simulink model "HEV_Ctrl_V1_1"  (R2018a)
settings: configuration reference "Config_Ctrl" (kept outside this file)
PreLoadFcn:
  | HEV_Ctrl_V1_PreLoad
undefined symbols (not defined in the file or in its folder): AstEnblEngSpdMin_H_K, AstEnblEngSpdMin_L_K, AstEnblSocMin_H_K, AstEnblSocMin_L_K, AstEnblVehSpdMin_H_K, AstEnblVehSpdMin_L_K, AstTrqCmpSOC_K2, AstTrqCmpSOC_X, AstTrqDstBase_K3, DifferentialGearRatio_K, DrvReqPropTrq_K3, DrvReqPropTrqMax_K, eHevCtrlMode, EngTrqMax_K2, EngTrqMax_K2x, HevCtrlEnbl_K, RchEnblEngSpdMin_H_K, RchEnblEngSpdMin_L_K, RchgEnblSocMax_H_K, RchgEnblSocMax_L_K, RchgTrqCmpSOC_K2, RchgTrqCmpSOC_X, RegnBrkCmpSOC_K2, RegnBrkCmpSOC_X, RegnBrkEnblBrkPdlMin_H_K, RegnBrkEnblBrkPdlMin_L_K, RegnBrkEnblSocMax_H_K, RegnBrkEnblSocMax_L_K, RegnBrkEnblVehSpdMin_H_K, RegnBrkEnblVehSpdMin_L_K, TransmissionGearRatio_K2
libraries: simulink x1
(part 1 of 2)
settings Model: DataDictionary=HEV_Ctrl_V1_Local_data.sldd  Creator=IAEC nishito  LastModifiedBy=E00026

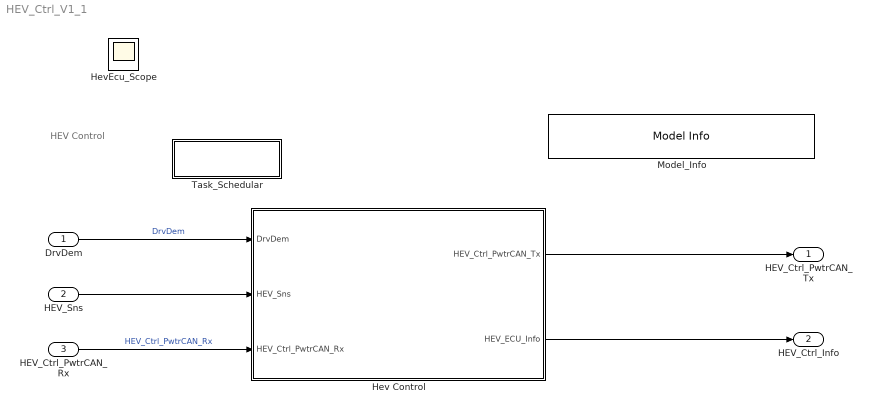
== system HEV_Ctrl_V1_1 ==
  note: HEV Control
  DrvDem : Inport  OutDataTypeStr=Bus: Driver_demand_Bus
      settings: AttributesFormatString=%<OutDataTypeStr>
  HEV_Sns : Inport  Port=2  OutDataTypeStr=Bus: HEV_sensor_Bus
      settings: AttributesFormatString=%<OutDataTypeStr>
  HEV_Ctrl_PwtrCAN_Rx : Inport  Port=3  OutDataTypeStr=Bus: HEV_Ctrl_PwtrCAN_Rx_Bus
      settings: AttributesFormatString=<%<OutDataTypeStr>>
  Hev Control : Subsystem
  Model_Info : simulink/Model-Wide Utilities/Model Info  Frame=on  DisplayStringWithTags=|  HorizontalTextAlignment=Left  LeftAlignmentValue=0.02
      | Version  %<ModelVersion>
      | LastModifided by %<LastModifiedBy>  Date %<LastModificationDate>
      | Description  %<Description>
  Task_Schedular : Subsystem
  HEV_Ctrl_PwtrCAN_Tx : Outport  OutDataTypeStr=Bus: HEV_Ctrl_PwtrCAN_Tx_Bus  VectorParamsAs1DForOutWhenUnconnected=off
      settings: AttributesFormatString=<%<OutDataTypeStr>>
  HEV_Ctrl_Info : Outport  Port=2  OutDataTypeStr=Bus: HEV_Ctrl_Info_Bus  VectorParamsAs1DForOutWhenUnconnected=off
      settings: AttributesFormatString=<%<OutDataTypeStr>>
  HevEcu_Scope : Scope
  wires:
  HEV_Ctrl_PwtrCAN_Rx/1 -> Hev Control/3(HEV_Ctrl_PwtrCAN_Rx)  "HEV_Ctrl_PwtrCAN_Rx"
  DrvDem/1 -> Hev Control/1(DrvDem)  "DrvDem"
  HEV_Sns/1 -> Hev Control/2(HEV_Sns)
  Hev Control/1(HEV_Ctrl_PwtrCAN_Tx) -> HEV_Ctrl_PwtrCAN_Tx/1
  Hev Control/2(HEV_ECU_Info) -> HEV_Ctrl_Info/1

== system HEV_Ctrl_V1_1/Hev Control ==
  DrvDem : Inport
  HEV_Sns : Inport  Port=2
  HEV_Ctrl_PwtrCAN_Rx : Inport  Port=3
  CAN_TX : Subsystem
  Energy Management : Subsystem
  Engine Control : Subsystem
  HevCtrl_In : Subsystem
  Idle Stop : Subsystem
  Info : Subsystem
  MotorControl : Subsystem
  HEV_Ctrl_PwtrCAN_Tx : Outport  VectorParamsAs1DForOutWhenUnconnected=off
  HEV_ECU_Info : Outport  Port=2  VectorParamsAs1DForOutWhenUnconnected=off
  wires:
  Energy Management/3(RegnBrkTrqMax) -> MotorControl/3(MaxRegnBrkTrq)
  DrvDem/1 -> HevCtrl_In/1(DrvDem)
  Energy Management/1(EngTrqReq) -> Engine Control/1(EngTrqReq_in)
  Energy Management/2(MtrTrqReq) -> MotorControl/2(MotTrqReq_in)
  HEV_Ctrl_PwtrCAN_Rx/1 -> HevCtrl_In/3(CAN)
  Engine Control/1(EngTrqReq) -> CAN_TX/2(EngTrqReq)
  MotorControl/1(MotTrqReq) -> CAN_TX/3(MotTrqReq)
  MotorControl/2(MotTrqWhl) -> CAN_TX/4(MotTrqWhl)
  MotorControl/3(MaxRegnBrkTrqWhl) -> CAN_TX/5(MaxRegnBrkTrqWhl)
  HEV_Sns/1 -> HevCtrl_In/2(HEV_Sns)
  CAN_TX/1(HEV_Ctrl_PwtrCAN_Tx) -> HEV_Ctrl_PwtrCAN_Tx/1
  Info/1(HEV_Ctrl_Info) -> HEV_ECU_Info/1
  HevCtrl_In/1(HevCtrl_In) -> Idle Stop/1(HevCtrl_In), Info/1(HevCtrl_In1), Engine Control/2(HevCtrlIn), MotorControl/1(HevCtrlIn), Energy Management/2(HevCtrl_In)
  Idle Stop/1(IdleStopCtrl) -> CAN_TX/1(IdleStopCtrl), Energy Management/1(IdleStopCtrl)

== system HEV_Ctrl_V1_1/Task_Schedular ==
  note: Task Schedular
  Task_Schedular_Chart : Stateflow chart  TreatAsAtomicUnit=on  SystemSampleTime=0.01
      settings: AttributesFormatString=<SampleTime = %<SystemSampleTime>>
  Terminator : Terminator
  tag scope: Evnt20ms=global
  wires:
  Task_Schedular_Chart/1(Evnt10ms()) -> Terminator/1
  Task_Schedular_Chart/2(Evnt20ms()) -> [Evnt20ms]

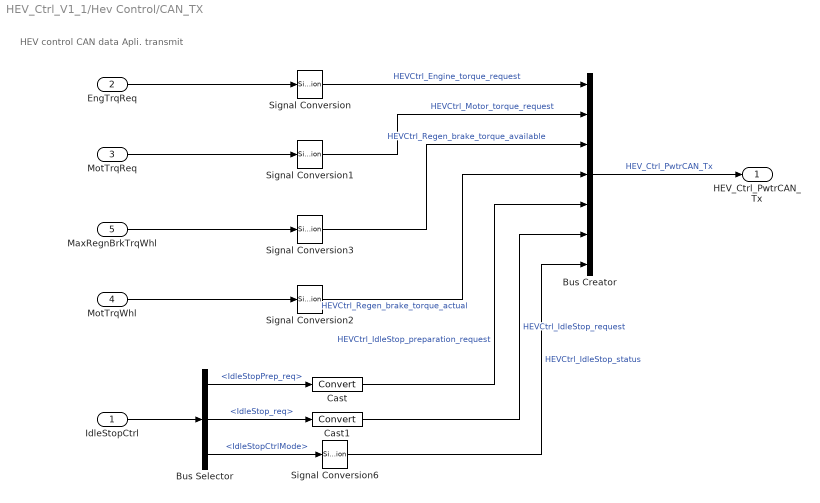
== system HEV_Ctrl_V1_1/Hev Control/CAN_TX ==
  note: HEV control CAN data Apli. transmit
  IdleStopCtrl : Inport
  EngTrqReq : Inport  Port=2
  MotTrqReq : Inport  Port=3
  MotTrqWhl : Inport  Port=4
  MaxRegnBrkTrqWhl : Inport  Port=5
  Bus Creator : BusCreator  Inputs=7  OutDataTypeStr=Bus: HEV_Ctrl_PwtrCAN_Tx_Bus
      settings: AttributesFormatString=<%<OutDataTypeStr>>
  Bus Selector : BusSelector  OutputSignals=IdleStopPrep_req,IdleStop_req,IdleStopCtrlMode
  Cast : DataTypeConversion
  Cast1 : DataTypeConversion
  Signal Conversion{,1..3,6} (5 alike) : SignalConversion  OverrideOpt=off
  HEV_Ctrl_PwtrCAN_Tx : Outport  VectorParamsAs1DForOutWhenUnconnected=off
  wires:
  Bus Creator/1 -> HEV_Ctrl_PwtrCAN_Tx/1  "HEV_Ctrl_PwtrCAN_Tx"
  MaxRegnBrkTrqWhl/1 -> Signal Conversion3/1
  MotTrqWhl/1 -> Signal Conversion2/1
  MotTrqReq/1 -> Signal Conversion1/1
  EngTrqReq/1 -> Signal Conversion/1
  Signal Conversion/1 -> Bus Creator/1  "HEVCtrl_Engine_torque_request"
  Signal Conversion1/1 -> Bus Creator/2  "HEVCtrl_Motor_torque_request"
  Signal Conversion3/1 -> Bus Creator/3  "HEVCtrl_Regen_brake_torque_available"
  Signal Conversion2/1 -> Bus Creator/4  "HEVCtrl_Regen_brake_torque_actual"
  Cast/1 -> Bus Creator/5  "HEVCtrl_IdleStop_preparation_request"
  Cast1/1 -> Bus Creator/6  "HEVCtrl_IdleStop_request"
  Signal Conversion6/1 -> Bus Creator/7  "HEVCtrl_IdleStop_status"
  IdleStopCtrl/1 -> Bus Selector/1
  Bus Selector/1 -> Cast/1  "<IdleStopPrep_req>"
  Bus Selector/2 -> Cast1/1  "<IdleStop_req>"
  Bus Selector/3 -> Signal Conversion6/1  "<IdleStopCtrlMode>"

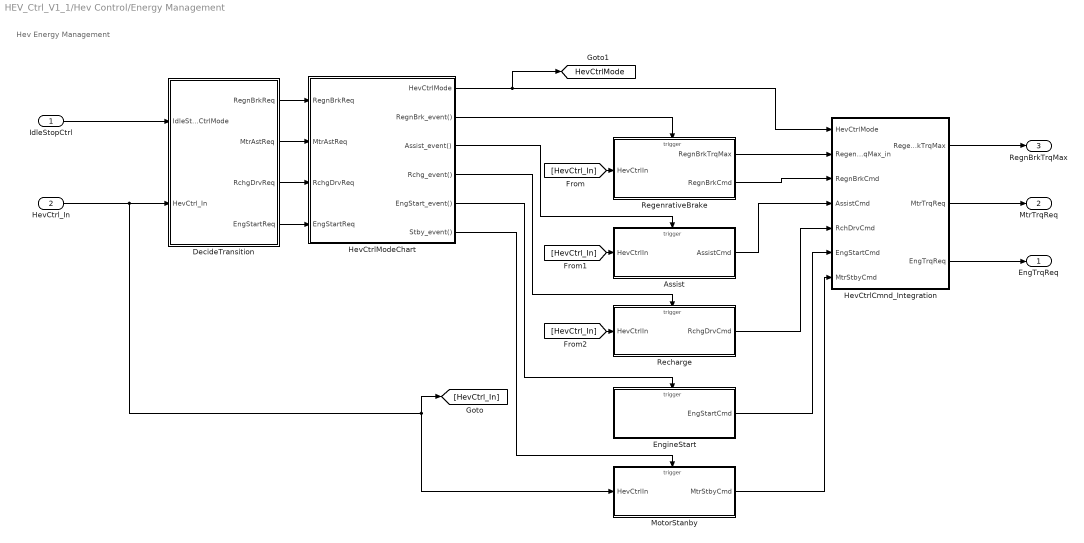
== system HEV_Ctrl_V1_1/Hev Control/Energy Management ==
  note: Hev Energy Management
  IdleStopCtrl : Inport
  HevCtrl_In : Inport  Port=2
  Assist : Subsystem  TreatAsAtomicUnit=on
  DecideTransition : Subsystem
  EngineStart : Subsystem  TreatAsAtomicUnit=on
  HevCtrlCmnd_Integration : Subsystem
  HevCtrlModeChart : Stateflow chart  TreatAsAtomicUnit=on
  MotorStanby : Subsystem  TreatAsAtomicUnit=on
  Recharge : Subsystem  TreatAsAtomicUnit=on
  RegenrativeBrake : Subsystem  TreatAsAtomicUnit=on
  EngTrqReq : Outport  VectorParamsAs1DForOutWhenUnconnected=off
  MtrTrqReq : Outport  Port=2  VectorParamsAs1DForOutWhenUnconnected=off
  RegnBrkTrqMax : Outport  Port=3  VectorParamsAs1DForOutWhenUnconnected=off
  tag scope: HevCtrlMode=global
  wires:
  DecideTransition/1(RegnBrkReq) -> HevCtrlModeChart/1(RegnBrkReq)
  DecideTransition/2(MtrAstReq) -> HevCtrlModeChart/2(MtrAstReq)
  DecideTransition/3(RchgDrvReq) -> HevCtrlModeChart/3(RchgDrvReq)
  HevCtrlModeChart/1(HevCtrlMode) -> [HevCtrlMode], HevCtrlCmnd_Integration/1(HevCtrlMode)
  HevCtrlModeChart/2(RegnBrk_event()) -> RegenrativeBrake/Trigger
  HevCtrlModeChart/3(Assist_event()) -> Assist/Trigger
  HevCtrlModeChart/4(Rchg_event()) -> Recharge/Trigger
  HevCtrlModeChart/5(EngStart_event()) -> EngineStart/Trigger
  RegenrativeBrake/1(RegnBrkTrqMax) -> HevCtrlCmnd_Integration/2(RegenBrkTrqMax_in)
  RegenrativeBrake/2(RegnBrkCmd) -> HevCtrlCmnd_Integration/3(RegnBrkCmd)
  Assist/1(AssistCmd) -> HevCtrlCmnd_Integration/4(AssistCmd)
  Recharge/1(RchgDrvCmd) -> HevCtrlCmnd_Integration/5(RchDrvCmd)
  EngineStart/1(EngStartCmd) -> HevCtrlCmnd_Integration/6(EngStartCmd)
  HevCtrlCmnd_Integration/2(MtrTrqReq) -> MtrTrqReq/1
  HevCtrlCmnd_Integration/3(EngTrqReq) -> EngTrqReq/1
  HevCtrlCmnd_Integration/1(RegenBrkTrqMax) -> RegnBrkTrqMax/1
  HevCtrl_In/1 -> DecideTransition/2(HevCtrl_In), MotorStanby/1(HevCtrlIn), [HevCtrl_In]
  [HevCtrl_In] -> RegenrativeBrake/1(HevCtrlIn)
  [HevCtrl_In] -> Assist/1(HevCtrlIn)
  [HevCtrl_In] -> Recharge/1(HevCtrlIn)
  HevCtrlModeChart/6(Stby_event()) -> MotorStanby/Trigger
  DecideTransition/4(EngStartReq) -> HevCtrlModeChart/4(EngStartReq)
  MotorStanby/1(MtrStbyCmd) -> HevCtrlCmnd_Integration/7(MtrStbyCmd)
  IdleStopCtrl/1 -> DecideTransition/1(IdleStopCtrlMode)

== system HEV_Ctrl_V1_1/Hev Control/Engine Control ==
  note: HEV Control Request to Engine Control
  EngTrqReq_in : Inport
  HevCtrlIn : Inport  Port=2
  Bus Selector2 : BusSelector  OutputSignals=EngineSpd
  K2_MaxEngTrq : Lookup  InputValues=EngTrqMax_K2x  Table=EngTrqMax_K2  LookUpMeth=Interpolation-Use End Values  SaturateOnIntegerOverflow=on
      settings: AttributesFormatString=<input=%<InputValues>>
  MaxLimit : MinMax  Inputs=2
  MinLimit : MinMax  Function=max  Inputs=2
  zero1 : Constant  Value=0
  EngTrqReq : Outport  VectorParamsAs1DForOutWhenUnconnected=off
  wires:
  HevCtrlIn/1 -> Bus Selector2/1
  EngTrqReq_in/1 -> MaxLimit/1
  MaxLimit/1 -> MinLimit/1
  K2_MaxEngTrq/1 -> MaxLimit/2
  MinLimit/1 -> EngTrqReq/1  "EngTrqReq"
  Bus Selector2/1 -> K2_MaxEngTrq/1  "<EngineSpd>"
  zero1/1 -> MinLimit/2

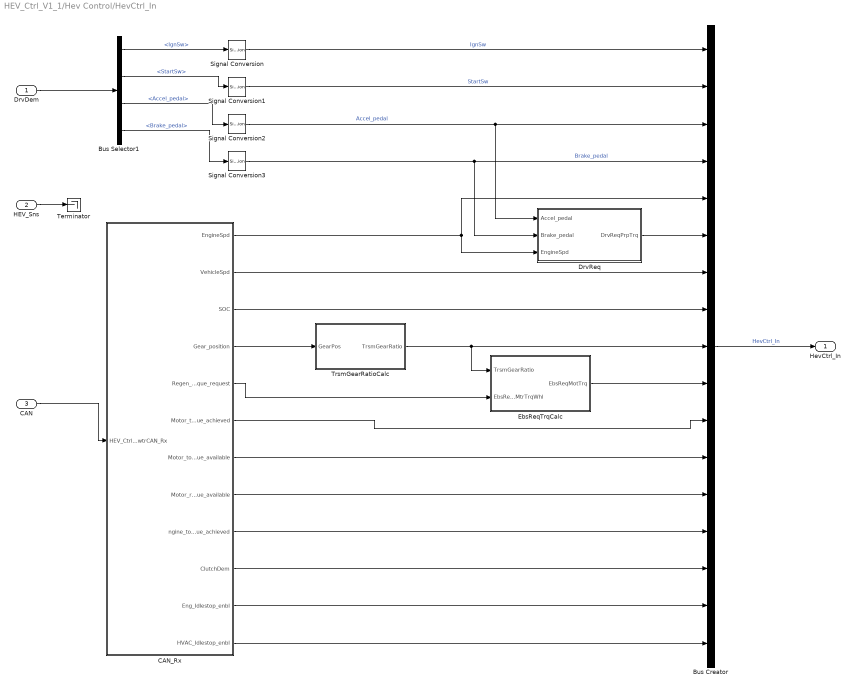
== system HEV_Ctrl_V1_1/Hev Control/HevCtrl_In ==
  DrvDem : Inport
  HEV_Sns : Inport  Port=2
  CAN : Inport  Port=3
  Bus Creator : BusCreator  Inputs=17
  Bus Selector1 : BusSelector  OutputSignals=IgnSw,StartSw,Accel_pedal,Brake_pedal
  CAN_Rx : Subsystem
  DrvReq : Subsystem
  EbsReqTrqCalc : Subsystem
  Signal Conversion{,1..3} (4 alike) : SignalConversion  OverrideOpt=off
  Terminator : Terminator
  TrsmGearRatioCalc : Subsystem
  HevCtrl_In : Outport  VectorParamsAs1DForOutWhenUnconnected=off
  wires:
  TrsmGearRatioCalc/1(TrsmGearRatio) -> Bus Creator/9, EbsReqTrqCalc/1(TrsmGearRatio)
  EbsReqTrqCalc/1(EbsReqMotTrq) -> Bus Creator/10
  HEV_Sns/1 -> Terminator/1
  Bus Creator/1 -> HevCtrl_In/1  "HevCtrl_In"
  DrvReq/1(DrvReqPrpTrq) -> Bus Creator/6
  DrvDem/1 -> Bus Selector1/1
  Signal Conversion/1 -> Bus Creator/1  "IgnSw"
  Signal Conversion1/1 -> Bus Creator/2  "StartSw"
  Signal Conversion2/1 -> DrvReq/1(Accel_pedal), Bus Creator/3  "Accel_pedal"
  Signal Conversion3/1 -> DrvReq/2(Brake_pedal), Bus Creator/4  "Brake_pedal"
  Bus Selector1/1 -> Signal Conversion/1  "<IgnSw>"
  Bus Selector1/2 -> Signal Conversion1/1  "<StartSw>"
  Bus Selector1/3 -> Signal Conversion2/1  "<Accel_pedal>"
  Bus Selector1/4 -> Signal Conversion3/1  "<Brake_pedal>"
  CAN_Rx/1(EngineSpd) -> DrvReq/3(EngineSpd), Bus Creator/5
  CAN/1 -> CAN_Rx/1(HEV_Ctrl_PwtrCAN_Rx)
  CAN_Rx/2(VehicleSpd) -> Bus Creator/7
  CAN_Rx/3(SOC) -> Bus Creator/8
  CAN_Rx/4(Gear_position) -> TrsmGearRatioCalc/1(GearPos)
  CAN_Rx/5(Regen_brake_torque_request) -> EbsReqTrqCalc/2(EbsReqMtrTrqWhl)
  CAN_Rx/6(Motor_torque_achieved) -> Bus Creator/11
  CAN_Rx/7(Motor_torque_available) -> Bus Creator/12
  CAN_Rx/8(Motor_regen_torque_available) -> Bus Creator/13
  CAN_Rx/9(ngine_torque_achieved) -> Bus Creator/14
  CAN_Rx/10(ClutchDem) -> Bus Creator/15
  CAN_Rx/11(Eng_Idlestop_enbl) -> Bus Creator/16
  CAN_Rx/12(HVAC_Idlestop_enbl) -> Bus Creator/17

== system HEV_Ctrl_V1_1/Hev Control/Idle Stop ==
  note: Idle Stop Control
  HevCtrl_In : Inport
  Bus Creator : BusCreator  Inputs=3
  Bus Selector2 : BusSelector  OutputSignals=VehicleSpd,Brake_pedal,Accel_pedal,SOC,Eng_Idlestop_enbl,HVAC_Idlestop_enbl,EngineSpd
  Idle_Stop_Control : ModelReference  ModelNameDialog=Idle_Stop_Control  SimulationMode=Normal  ModelReferenceVersion=1.0.4  TriggerPortName=Trigger  TriggerPortTriggerType=function-call  TriggerPortStatesWhenEnabling=held
  IdleStopCtrl : Outport  VectorParamsAs1DForOutWhenUnconnected=off
  wires:
  HevCtrl_In/1 -> Bus Selector2/1
  Bus Creator/1 -> IdleStopCtrl/1  "IdleStopCtrl"
  Bus Selector2/1 -> Idle_Stop_Control/1  "<VehicleSpd>"
  Bus Selector2/2 -> Idle_Stop_Control/2  "<Brake_pedal>"
  Bus Selector2/3 -> Idle_Stop_Control/3  "<Accel_pedal>"
  Bus Selector2/4 -> Idle_Stop_Control/4  "<SOC>"
  Bus Selector2/5 -> Idle_Stop_Control/5  "<Eng_Idlestop_enbl>"
  Bus Selector2/6 -> Idle_Stop_Control/6  "<HVAC_Idlestop_enbl>"
  Bus Selector2/7 -> Idle_Stop_Control/7  "<EngineSpd>"
  Idle_Stop_Control/1 -> Bus Creator/1  "IdleStopCtrlMode"
  Idle_Stop_Control/2 -> Bus Creator/2  "IdleStopPrep_req"
  Idle_Stop_Control/3 -> Bus Creator/3  "IdleStop_req"
  [Evnt20ms] -> Idle_Stop_Control/Trigger

== system HEV_Ctrl_V1_1/Hev Control/Info ==
  HevCtrl_In1 : Inport
  Bus Creator : BusCreator  Inputs=2  OutDataTypeStr=Bus: HEV_Ctrl_Info_Bus
      settings: AttributesFormatString=%<OutDataTypeStr>
  Bus Selector : BusSelector  OutputSignals=DrvReqPrpTrq
  Data Type Conversion : DataTypeConversion  OutDataTypeStr=double
  Signal Conversion : SignalConversion  OverrideOpt=off
  HEV_Ctrl_Info : Outport  VectorParamsAs1DForOutWhenUnconnected=off
  wires:
  HevCtrl_In1/1 -> Bus Selector/1
  Bus Creator/1 -> HEV_Ctrl_Info/1  "HEV_Ctrl_Info"
  Bus Selector/1 -> Signal Conversion/1  "<DrvReqPrpTrq>"
  [HevCtrlMode] -> Data Type Conversion/1
  Data Type Conversion/1 -> Bus Creator/2  "HEVCtrl_HevCtrlMode"
  Signal Conversion/1 -> Bus Creator/1  "HEVCtrl_DrvReqPrpTrq"

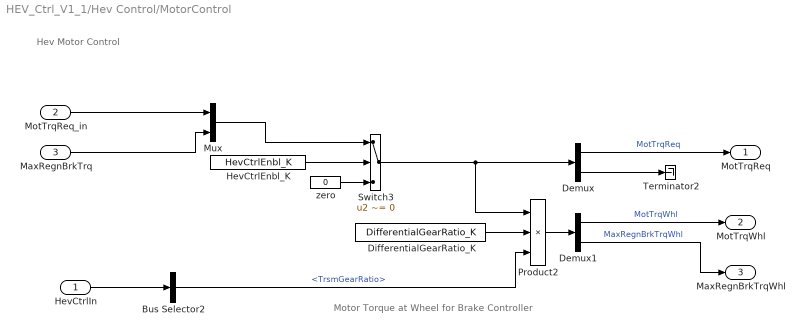
== system HEV_Ctrl_V1_1/Hev Control/MotorControl ==
  note: Motor Torque at Wheel for Brake Controller
  note: Hev Motor Control
  HevCtrlIn : Inport
  MotTrqReq_in : Inport  Port=2
  MaxRegnBrkTrq : Inport  Port=3
  Bus Selector2 : BusSelector  OutputSignals=TrsmGearRatio
  Demux : Demux  Outputs=2
  Demux1 : Demux  Outputs=2
  DifferentialGearRatio_K : Constant  Value=DifferentialGearRatio_K
  HevCtrlEnbl_K : Constant  Value=HevCtrlEnbl_K
  Mux : Mux  Inputs=2
  Product2 : Product  Inputs=3  RndMeth=Zero
  Switch3 : Switch  Criteria=u2 ~= 0  Threshold=0.5  SaturateOnIntegerOverflow=on
      settings: AttributesFormatString=<%<Criteria>>
  Terminator2 : Terminator
  zero : Constant  Value=0
  MotTrqReq : Outport  VectorParamsAs1DForOutWhenUnconnected=off
  MotTrqWhl : Outport  Port=2  VectorParamsAs1DForOutWhenUnconnected=off
  MaxRegnBrkTrqWhl : Outport  Port=3  VectorParamsAs1DForOutWhenUnconnected=off
  wires:
  Demux/2 -> Terminator2/1
  Demux1/2 -> MaxRegnBrkTrqWhl/1  "MaxRegnBrkTrqWhl"
  Product2/1 -> Demux1/1
  Demux/1 -> MotTrqReq/1  "MotTrqReq"
  Demux1/1 -> MotTrqWhl/1  "MotTrqWhl"
  Bus Selector2/1 -> Product2/3  "<TrsmGearRatio>"
  MotTrqReq_in/1 -> Mux/1
  HevCtrlEnbl_K/1 -> Switch3/2
  zero/1 -> Switch3/3
  Switch3/1 -> Product2/1, Demux/1
  DifferentialGearRatio_K/1 -> Product2/2
  HevCtrlIn/1 -> Bus Selector2/1
  Mux/1 -> Switch3/1
  MaxRegnBrkTrq/1 -> Mux/2

== system HEV_Ctrl_V1_1/Hev Control/Energy Management/Assist ==
  note: Assist
  HevCtrlIn : Inport
  Trigger : TriggerPort  TriggerType=function-call  VariantControl=Variant
  Bus Creator : BusCreator  Inputs=2
  Bus Selector : BusSelector  OutputSignals=DrvReqPrpTrq,Motor_torque_available,EngineSpd,SOC
  MotorAssist : Subsystem
  AssistCmd : Outport  VectorParamsAs1DForOutWhenUnconnected=off
  wires:
  HevCtrlIn/1 -> Bus Selector/1
  Bus Creator/1 -> AssistCmd/1  "AssistCmd"
  MotorAssist/1(MtrTrqReq) -> Bus Creator/1
  MotorAssist/2(EngTrqReq) -> Bus Creator/2
  Bus Selector/1 -> MotorAssist/1(DrvReqTrq)  "<DrvReqPrpTrq>"
  Bus Selector/2 -> MotorAssist/2(MtrPrpTrqMax)  "<Motor_torque_available>"
  Bus Selector/3 -> MotorAssist/3(EngSpd)  "<EngineSpd>"
  Bus Selector/4 -> MotorAssist/4(BatSoc)  "<SOC>"

== system HEV_Ctrl_V1_1/Hev Control/Energy Management/DecideTransition ==
  note: Decide Transition
  IdleStopCtrlMode : Inport
  HevCtrl_In : Inport  Port=2
  Assist : Subsystem
  Bus Selector : BusSelector  OutputSignals=DrvReqPrpTrq,VehicleSpd,EngineSpd,Brake_pedal,SOC
  Bus Selector1 : BusSelector  OutputSignals=DrvReqPrpTrq,EngineSpd,Brake_pedal,SOC
  Bus Selector2 : BusSelector  OutputSignals=VehicleSpd,Brake_pedal,SOC,EngineSpd
  Bus Selector3 : BusSelector  OutputSignals=IgnSw,StartSw,EngineSpd
  Bus Selector4 : BusSelector  OutputSignals=IdleStopCtrlMode
  EngineStart : Subsystem
  RchgDrvJdg : Subsystem
  RegBrake : Subsystem
  RegnBrkReq : Outport  VectorParamsAs1DForOutWhenUnconnected=off
  MtrAstReq : Outport  Port=2  VectorParamsAs1DForOutWhenUnconnected=off
  RchgDrvReq : Outport  Port=3  VectorParamsAs1DForOutWhenUnconnected=off
  EngStartReq : Outport  Port=4  VectorParamsAs1DForOutWhenUnconnected=off
  wires:
  Assist/1(MtrAstReq) -> MtrAstReq/1
  RegBrake/1(RegnBrkReqFlag) -> RegnBrkReq/1
  RchgDrvJdg/1(RchgDrvReq) -> RchgDrvReq/1
  HevCtrl_In/1 -> Bus Selector2/1, Bus Selector/1, Bus Selector3/1, Bus Selector1/1
  Bus Selector2/1 -> RegBrake/1(Vehicle_speed)  "<VehicleSpd>"
  Bus Selector2/2 -> RegBrake/2(Brake_pedal)  "<Brake_pedal>"
  Bus Selector2/3 -> RegBrake/3(Bat_soc)  "<SOC>"
  Bus Selector/2 -> Assist/2(VehSpd)  "<VehicleSpd>"
  Bus Selector/3 -> Assist/3(EngSpd)  "<EngineSpd>"
  Bus Selector/4 -> Assist/4(Brake_pedal)  "<Brake_pedal>"
  Bus Selector/5 -> Assist/5(BatSoc)  "<SOC>"
  Bus Selector1/2 -> RchgDrvJdg/2(EngSpd)  "<EngineSpd>"
  Bus Selector1/3 -> RchgDrvJdg/3(Brake_pedal)  "<Brake_pedal>"
  Bus Selector1/4 -> RchgDrvJdg/4(BatSoc)  "<SOC>"
  Bus Selector/1 -> Assist/1(DrvReqTrq)  "<DrvReqPrpTrq>"
  Bus Selector1/1 -> RchgDrvJdg/1(DrvReqTrq)  "<DrvReqPrpTrq>"
  Bus Selector2/4 -> RegBrake/4(EngSpd)  "<EngineSpd>"
  Bus Selector3/1 -> EngineStart/1(IgnSw)  "<IgnSw>"
  Bus Selector3/2 -> EngineStart/2(StartSw)  "<StartSw>"
  Bus Selector3/3 -> EngineStart/3(EngineSpd)  "<EngineSpd>"
  EngineStart/1(EngStartReq) -> EngStartReq/1
  IdleStopCtrlMode/1 -> Bus Selector4/1
  Bus Selector4/1 -> EngineStart/4(IdleStopCtrlMode)  "<IdleStopCtrlMode>"

== system HEV_Ctrl_V1_1/Hev Control/Energy Management/EngineStart ==
  note: Engine Start
  Trigger : TriggerPort  TriggerType=function-call  VariantControl=Variant
  Bus Creator : BusCreator  Inputs=2
  EngineStartTrq : Constant  Value=50
  zero : Constant  Value=0
  EngStartCmd : Outport  VectorParamsAs1DForOutWhenUnconnected=off
  wires:
  zero/1 -> Bus Creator/2  "EngTrqReq"
  Bus Creator/1 -> EngStartCmd/1  "EngStartCmd"
  EngineStartTrq/1 -> Bus Creator/1  "MtrTrqReq"

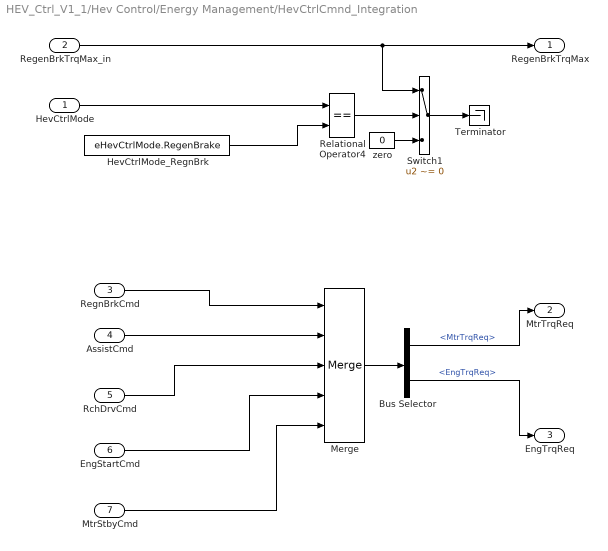
== system HEV_Ctrl_V1_1/Hev Control/Energy Management/HevCtrlCmnd_Integration ==
  HevCtrlMode : Inport
  RegenBrkTrqMax_in : Inport  Port=2
  RegnBrkCmd : Inport  Port=3
  AssistCmd : Inport  Port=4
  RchDrvCmd : Inport  Port=5
  EngStartCmd : Inport  Port=6
  MtrStbyCmd : Inport  Port=7
  Bus Selector : BusSelector  OutputSignals=MtrTrqReq,EngTrqReq
  HevCtrlMode_RegnBrk : Constant  Value=eHevCtrlMode.RegenBrake  OutDataTypeStr=Enum: eHevCtrlMode
  Merge : Merge  Inputs=5
  Relational Operator4 : RelationalOperator  Operator===  OutDataTypeStr=boolean  RndMeth=Nearest
  Switch1 : Switch  Criteria=u2 ~= 0  Threshold=0.5  SaturateOnIntegerOverflow=on
      settings: AttributesFormatString=<%<Criteria>>
  Terminator : Terminator
  zero : Constant  Value=0
  RegenBrkTrqMax : Outport  VectorParamsAs1DForOutWhenUnconnected=off
  MtrTrqReq : Outport  Port=2  VectorParamsAs1DForOutWhenUnconnected=off
  EngTrqReq : Outport  Port=3  VectorParamsAs1DForOutWhenUnconnected=off
  wires:
  Merge/1 -> Bus Selector/1
  zero/1 -> Switch1/3
  HevCtrlMode/1 -> Relational Operator4/1
  RegenBrkTrqMax_in/1 -> Switch1/1, RegenBrkTrqMax/1
  RegnBrkCmd/1 -> Merge/1
  Bus Selector/1 -> MtrTrqReq/1  "<MtrTrqReq>"
  AssistCmd/1 -> Merge/2
  Bus Selector/2 -> EngTrqReq/1  "<EngTrqReq>"
  RchDrvCmd/1 -> Merge/3
  EngStartCmd/1 -> Merge/4
  HevCtrlMode_RegnBrk/1 -> Relational Operator4/2
  Relational Operator4/1 -> Switch1/2
  Switch1/1 -> Terminator/1
  MtrStbyCmd/1 -> Merge/5

== system HEV_Ctrl_V1_1/Hev Control/Energy Management/MotorStanby ==
  note: Motor Standby
  HevCtrlIn : Inport
  Trigger : TriggerPort  TriggerType=function-call  VariantControl=Variant
  Bus Creator : BusCreator  Inputs=2
  Bus Selector : BusSelector  OutputSignals=DrvReqPrpTrq,EngineSpd,ClutchDem
  Constant2 : Constant  Value=200
  Constant4 : Constant  Value=0.5
  EngTrqZero : Constant  Value=0
  Logical Operator : Logic  AllPortsSameDT=off  OutDataTypeStr=boolean
  Relational Operator1 : RelationalOperator  Operator=>  OutDataTypeStr=boolean  RndMeth=Nearest
  Relational Operator4 : RelationalOperator  Operator=>  OutDataTypeStr=boolean  RndMeth=Nearest
  Switch : Switch  Criteria=u2 ~= 0  Threshold=0.5  SaturateOnIntegerOverflow=on
      settings: AttributesFormatString=<%<Criteria>>
  zero : Constant  Value=0
  MtrStbyCmd : Outport  VectorParamsAs1DForOutWhenUnconnected=off
  wires:
  Bus Selector/1 -> Switch/1  "<DrvReqPrpTrq>"
  zero/1 -> Bus Creator/1  "MtrTrqReq"
  Bus Creator/1 -> MtrStbyCmd/1  "MtrStbyCmd"
  Switch/1 -> Bus Creator/2  "EngTrqReq"
  HevCtrlIn/1 -> Bus Selector/1
  Bus Selector/2 -> Relational Operator1/1  "<EngineSpd>"
  Relational Operator4/1 -> Logical Operator/2
  Relational Operator1/1 -> Logical Operator/1
  Constant2/1 -> Relational Operator1/2
  Logical Operator/1 -> Switch/2
  Bus Selector/3 -> Relational Operator4/1  "<ClutchDem>"
  Constant4/1 -> Relational Operator4/2
  EngTrqZero/1 -> Switch/3

== system HEV_Ctrl_V1_1/Hev Control/Energy Management/Recharge ==
  note: Recharge
  HevCtrlIn : Inport
  Trigger : TriggerPort  TriggerType=function-call  VariantControl=Variant
  Bus Creator : BusCreator  Inputs=2
  Bus Selector : BusSelector  OutputSignals=DrvReqPrpTrq,EngineSpd,Motor_regen_torque_available,SOC
  Recharge : Subsystem
  RchgDrvCmd : Outport  VectorParamsAs1DForOutWhenUnconnected=off
  wires:
  Recharge/2(EngTrqReq) -> Bus Creator/2
  Bus Creator/1 -> RchgDrvCmd/1  "RchgDrvCmd"
  HevCtrlIn/1 -> Bus Selector/1
  Recharge/1(MtrTrqReq) -> Bus Creator/1
  Bus Selector/1 -> Recharge/1(DrvReqTrq)  "<DrvReqPrpTrq>"
  Bus Selector/2 -> Recharge/2(EngSpd)  "<EngineSpd>"
  Bus Selector/3 -> Recharge/3(MtrRgnTrqMax)  "<Motor_regen_torque_available>"
  Bus Selector/4 -> Recharge/4(BatSOC)  "<SOC>"

== system HEV_Ctrl_V1_1/Hev Control/Energy Management/RegenrativeBrake ==
  note: Regenerative Brake
  HevCtrlIn : Inport
  Trigger : TriggerPort  TriggerType=function-call  VariantControl=Variant
  Bus Creator : BusCreator  Inputs=2
  Bus Selector2 : BusSelector  OutputSignals=Motor_torque_available,SOC,EbsReq_RegnBrkTrq
  Regenerative Brake : Subsystem
  zero : Constant  Value=0
  RegnBrkTrqMax : Outport  VectorParamsAs1DForOutWhenUnconnected=off
  RegnBrkCmd : Outport  Port=2  VectorParamsAs1DForOutWhenUnconnected=off
  wires:
  Regenerative Brake/2(RegnBrkTrqMax) -> RegnBrkTrqMax/1
  HevCtrlIn/1 -> Bus Selector2/1
  zero/1 -> Bus Creator/2  "EngTrqReq"
  Bus Creator/1 -> RegnBrkCmd/1  "RegnBrkCmd"
  Regenerative Brake/1(MtrTrqReq) -> Bus Creator/1
  Bus Selector2/1 -> Regenerative Brake/1(MaxRegnTrq)  "<Motor_torque_available>"
  Bus Selector2/2 -> Regenerative Brake/2(BattSOC)  "<SOC>"
  Bus Selector2/3 -> Regenerative Brake/3(EbsReqMtrTrq)  "<EbsReq_RegnBrkTrq>"

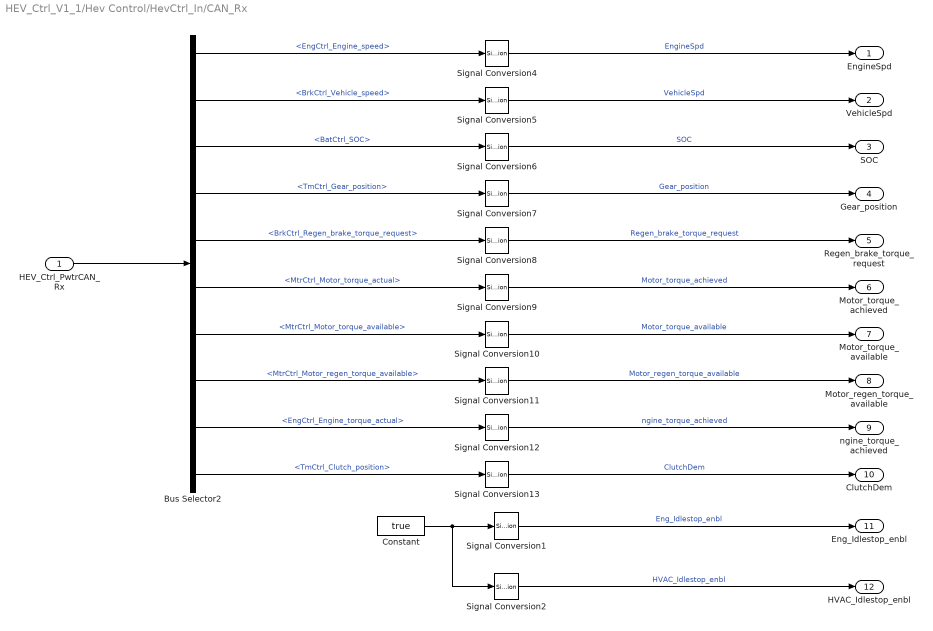
== system HEV_Ctrl_V1_1/Hev Control/HevCtrl_In/CAN_Rx ==
  HEV_Ctrl_PwtrCAN_Rx : Inport
  Bus Selector2 : BusSelector  OutputSignals=EngCtrl_Engine_speed,BrkCtrl_Vehicle_speed,BatCtrl_SOC,TmCtrl_Gear_position,BrkCtrl_Regen_brake_torque_request,MtrCtrl_Motor_torque_actual,MtrCtrl_Motor_torque_available,MtrCtrl_Motor_regen_torque_available,EngCtrl_Engine_torque_actual,TmCtrl_Clutch_position
  Constant : Constant  Value=true
  Signal Conversion{1..2,4..13} (12 alike) : SignalConversion  OverrideOpt=off
  EngineSpd : Outport  VectorParamsAs1DForOutWhenUnconnected=off
  VehicleSpd : Outport  Port=2  VectorParamsAs1DForOutWhenUnconnected=off
  SOC : Outport  Port=3  VectorParamsAs1DForOutWhenUnconnected=off
  Gear_position : Outport  Port=4  VectorParamsAs1DForOutWhenUnconnected=off
  Regen_brake_torque_request : Outport  Port=5  VectorParamsAs1DForOutWhenUnconnected=off
  Motor_torque_achieved : Outport  Port=6  VectorParamsAs1DForOutWhenUnconnected=off
  Motor_torque_available : Outport  Port=7  VectorParamsAs1DForOutWhenUnconnected=off
  Motor_regen_torque_available : Outport  Port=8  VectorParamsAs1DForOutWhenUnconnected=off
  ngine_torque_achieved : Outport  Port=9  VectorParamsAs1DForOutWhenUnconnected=off
  ClutchDem : Outport  Port=10  VectorParamsAs1DForOutWhenUnconnected=off
  Eng_Idlestop_enbl : Outport  Port=11  VectorParamsAs1DForOutWhenUnconnected=off
  HVAC_Idlestop_enbl : Outport  Port=12  VectorParamsAs1DForOutWhenUnconnected=off
  wires:
  Bus Selector2/3 -> Signal Conversion6/1  "<BatCtrl_SOC>"
  Bus Selector2/10 -> Signal Conversion13/1  "<TmCtrl_Clutch_position>"
  Signal Conversion13/1 -> ClutchDem/1  "ClutchDem"
  Bus Selector2/7 -> Signal Conversion10/1  "<MtrCtrl_Motor_torque_available>"
  Bus Selector2/1 -> Signal Conversion4/1  "<EngCtrl_Engine_speed>"
  Bus Selector2/5 -> Signal Conversion8/1  "<BrkCtrl_Regen_brake_torque_request>"
  Signal Conversion11/1 -> Motor_regen_torque_available/1  "Motor_regen_torque_available"
  Signal Conversion12/1 -> ngine_torque_achieved/1  "ngine_torque_achieved"
  Bus Selector2/8 -> Signal Conversion11/1  "<MtrCtrl_Motor_regen_torque_available>"
  Bus Selector2/2 -> Signal Conversion5/1  "<BrkCtrl_Vehicle_speed>"
  Signal Conversion7/1 -> Gear_position/1  "Gear_position"
  Bus Selector2/6 -> Signal Conversion9/1  "<MtrCtrl_Motor_torque_actual>"
  HEV_Ctrl_PwtrCAN_Rx/1 -> Bus Selector2/1
  Bus Selector2/9 -> Signal Conversion12/1  "<EngCtrl_Engine_torque_actual>"
  Bus Selector2/4 -> Signal Conversion7/1  "<TmCtrl_Gear_position>"
  Signal Conversion8/1 -> Regen_brake_torque_request/1  "Regen_brake_torque_request"
  Signal Conversion5/1 -> VehicleSpd/1  "VehicleSpd"
  Signal Conversion10/1 -> Motor_torque_available/1  "Motor_torque_available"
  Signal Conversion9/1 -> Motor_torque_achieved/1  "Motor_torque_achieved"
  Signal Conversion4/1 -> EngineSpd/1  "EngineSpd"
  Signal Conversion6/1 -> SOC/1  "SOC"
  Signal Conversion1/1 -> Eng_Idlestop_enbl/1  "Eng_Idlestop_enbl"
  Constant/1 -> Signal Conversion2/1, Signal Conversion1/1
  Signal Conversion2/1 -> HVAC_Idlestop_enbl/1  "HVAC_Idlestop_enbl"

== system HEV_Ctrl_V1_1/Hev Control/HevCtrl_In/DrvReq ==
  note: Hev Control Driver Request
  note: The brake operation is higher priority than the accel operation
  Accel_pedal : Inport
  Brake_pedal : Inport  Port=2
  EngineSpd : Inport  Port=3
  Constant : Constant  Value=0.1
  DrvReqPropTrqMax_K : Constant  Value=DrvReqPropTrqMax_K
  DrvReqPropTrq_K3 : Lookup2D  RowIndex=DrvReqPropTrq_K3y  ColumnIndex=DrvReqPropTrq_K3x  Table=DrvReqPropTrq_K3  LookUpMeth=Interpolation-Use End Values  SaturateOnIntegerOverflow=on
      settings: AttributesFormatString=<row=%<RowIndex>>\n<column=%<ColumnIndex>>
  Gain_inv_percent : Gain  Gain=0.01
  MaxLimit : MinMax  Inputs=2
  Mul : Product
  Relational Operator : RelationalOperator  Operator=<  OutDataTypeStr=boolean  RndMeth=Nearest
  Switch1 : Switch  Criteria=u2 ~= 0  Threshold=0.5  SaturateOnIntegerOverflow=on
      settings: AttributesFormatString=<%<Criteria>>
  zero : Constant  Value=0
  DrvReqPrpTrq : Outport  VectorParamsAs1DForOutWhenUnconnected=off
  wires:
  Mul/1 -> Switch1/1, MaxLimit/2
  EngineSpd/1 -> DrvReqPropTrq_K3/2
  Brake_pedal/1 -> Relational Operator/1
  Constant/1 -> Relational Operator/2
  Relational Operator/1 -> Switch1/2
  zero/1 -> MaxLimit/1
  MaxLimit/1 -> Switch1/3
  Switch1/1 -> DrvReqPrpTrq/1  "DrvReqPrpTrq"
  DrvReqPropTrqMax_K/1 -> Mul/1
  DrvReqPropTrq_K3/1 -> Gain_inv_percent/1
  Gain_inv_percent/1 -> Mul/2
  Accel_pedal/1 -> DrvReqPropTrq_K3/1

== system HEV_Ctrl_V1_1/Hev Control/HevCtrl_In/EbsReqTrqCalc ==
  note: BrakeTorque @Wheel Positive <--|--> @Crank Negative
  note: EBS Brake Torque conversion from @wheel to @crank
  TrsmGearRatio : Inport
  EbsReqMtrTrqWhl : Inport  Port=2
  DifferentialGearRatio_K : Constant  Value=DifferentialGearRatio_K
  Gain2 : Gain  Gain=-1
  Product1 : Product  Inputs=*//  RndMeth=Zero
  EbsReqMotTrq : Outport  VectorParamsAs1DForOutWhenUnconnected=off
  wires:
  Gain2/1 -> EbsReqMotTrq/1  "EbsReq_RegnBrkTrq"
  Product1/1 -> Gain2/1  "EbsReqMtrTrq"
  DifferentialGearRatio_K/1 -> Product1/3
  TrsmGearRatio/1 -> Product1/2
  EbsReqMtrTrqWhl/1 -> Product1/1

== system HEV_Ctrl_V1_1/Hev Control/HevCtrl_In/TrsmGearRatioCalc ==
  note: if GearPos == 0(Neutral) TrsmGearRatio is old value
  note: Transmission Gear Ratio Calc.
  GearPos : Inport
  Relational Operator1 : RelationalOperator  OutDataTypeStr=boolean  RndMeth=Nearest
  Selector : Selector  InputPortWidth=TransmissionGearPosMax_K  IndexOptions=Index vector (port)  Indices=[1 3]  OutputSizes=1
  Switch1 : Switch  Criteria=u2 ~= 0  Threshold=0.5  SaturateOnIntegerOverflow=on
      settings: AttributesFormatString=<%<Criteria>>
  TransmissionGearRatio_K2 : Constant  Value=TransmissionGearRatio_K2
  Unit Delay : UnitDelay  InitialCondition=1  SampleTime=-1  HasFrameUpgradeWarning=on
      settings: AttributesFormatString=<initial=%<X0>>\n<tsample=%<SampleTime>>
  one : Constant
  TrsmGearRatio : Outport  VectorParamsAs1DForOutWhenUnconnected=off
  wires:
  Selector/1 -> TrsmGearRatio/1  "TrsmGearRatio"
  GearPos/1 -> Switch1/1, Relational Operator1/1
  Relational Operator1/1 -> Switch1/2
  Unit Delay/1 -> Switch1/3
  one/1 -> Relational Operator1/2
  Switch1/1 -> Selector/2, Unit Delay/1
  TransmissionGearRatio_K2/1 -> Selector/1

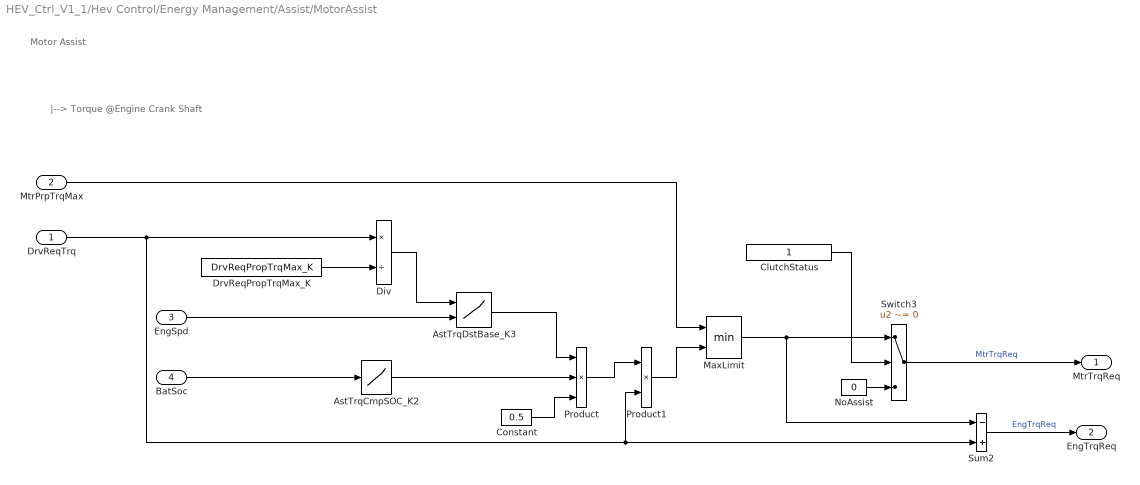
== system HEV_Ctrl_V1_1/Hev Control/Energy Management/Assist/MotorAssist ==
  note: |--> Torque @Engine Crank Shaft
  note: Motor Assist
  DrvReqTrq : Inport
  MtrPrpTrqMax : Inport  Port=2
  EngSpd : Inport  Port=3
  BatSoc : Inport  Port=4
  AstTrqCmpSOC_K2 : Lookup  InputValues=AstTrqCmpSOC_X  Table=AstTrqCmpSOC_K2  LookUpMeth=Interpolation-Use End Values  SaturateOnIntegerOverflow=on
      settings: AttributesFormatString=<input=%<InputValues>>
  AstTrqDstBase_K3 : Lookup2D  RowIndex=AstTrqDstBase_Y  ColumnIndex=AstTrqDstBase_X  Table=AstTrqDstBase_K3  LookUpMeth=Interpolation-Use End Values  SaturateOnIntegerOverflow=on
      settings: AttributesFormatString=<row=%<RowIndex>>\n<column=%<ColumnIndex>>
  ClutchStatus : Constant
  Constant : Constant  Value=0.5
  Div : Product  Inputs=*/
  DrvReqPropTrqMax_K : Constant  Value=DrvReqPropTrqMax_K
  MaxLimit : MinMax  Inputs=2
  NoAssist : Constant  Value=0
  Product : Product  Inputs=3  RndMeth=Zero
  Product1 : Product  RndMeth=Zero
  Sum2 : Sum  Inputs=-+
  Switch3 : Switch  Criteria=u2 ~= 0  Threshold=0.5  SaturateOnIntegerOverflow=on
      settings: AttributesFormatString=<%<Criteria>>
  MtrTrqReq : Outport  VectorParamsAs1DForOutWhenUnconnected=off
  EngTrqReq : Outport  Port=2  VectorParamsAs1DForOutWhenUnconnected=off
  wires:
  NoAssist/1 -> Switch3/3
  Switch3/1 -> MtrTrqReq/1  "MtrTrqReq"
  AstTrqCmpSOC_K2/1 -> Product/2
  Product/1 -> Product1/1
  MaxLimit/1 -> Switch3/1, Sum2/1
  Sum2/1 -> EngTrqReq/1  "EngTrqReq"
  MtrPrpTrqMax/1 -> MaxLimit/1
  ClutchStatus/1 -> Switch3/2
  EngSpd/1 -> AstTrqDstBase_K3/2
  DrvReqTrq/1 -> Div/1, Sum2/2, Product1/2
  DrvReqPropTrqMax_K/1 -> Div/2
  Div/1 -> AstTrqDstBase_K3/1
  AstTrqDstBase_K3/1 -> Product/1
  BatSoc/1 -> AstTrqCmpSOC_K2/1
  Product1/1 -> MaxLimit/2
  Constant/1 -> Product/3

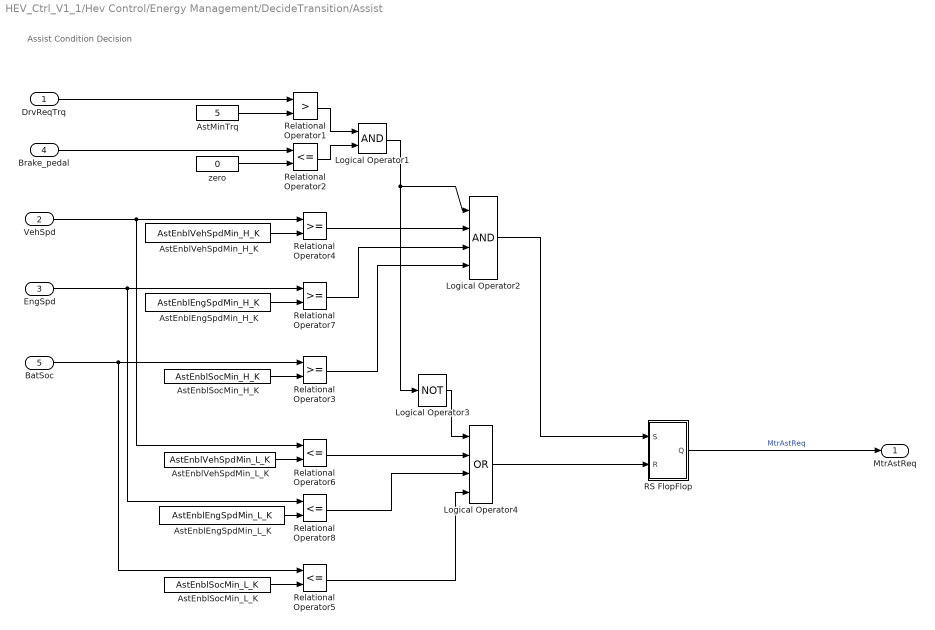
== system HEV_Ctrl_V1_1/Hev Control/Energy Management/DecideTransition/Assist ==
  note: Assist Condition Decision
  DrvReqTrq : Inport
  VehSpd : Inport  Port=2
  EngSpd : Inport  Port=3
  Brake_pedal : Inport  Port=4
  BatSoc : Inport  Port=5
  AstEnblEngSpdMin_H_K : Constant  Value=AstEnblEngSpdMin_H_K
  AstEnblEngSpdMin_L_K : Constant  Value=AstEnblEngSpdMin_L_K
  AstEnblSocMin_H_K : Constant  Value=AstEnblSocMin_H_K
  AstEnblSocMin_L_K : Constant  Value=AstEnblSocMin_L_K
  AstEnblVehSpdMin_H_K : Constant  Value=AstEnblVehSpdMin_H_K
  AstEnblVehSpdMin_L_K : Constant  Value=AstEnblVehSpdMin_L_K
  AstMinTrq : Constant  Value=5
  Logical Operator1 : Logic  AllPortsSameDT=off  OutDataTypeStr=boolean
  Logical Operator2 : Logic  Inputs=4  AllPortsSameDT=off  OutDataTypeStr=boolean
  Logical Operator3 : Logic  Operator=NOT  AllPortsSameDT=off  OutDataTypeStr=boolean
  Logical Operator4 : Logic  Operator=OR  Inputs=4  AllPortsSameDT=off  OutDataTypeStr=boolean
  RS FlopFlop : Subsystem
  Relational Operator1 : RelationalOperator  Operator=>  OutDataTypeStr=boolean  RndMeth=Nearest
  Relational Operator{2,5..6,8} (4 alike) : RelationalOperator  Operator=<=  OutDataTypeStr=boolean  RndMeth=Nearest
  Relational Operator3 : RelationalOperator  OutDataTypeStr=boolean  RndMeth=Nearest
  Relational Operator4 : RelationalOperator  OutDataTypeStr=boolean  RndMeth=Nearest
  Relational Operator7 : RelationalOperator  OutDataTypeStr=boolean  RndMeth=Nearest
  zero : Constant  Value=0
  MtrAstReq : Outport  VectorParamsAs1DForOutWhenUnconnected=off
  wires:
  Logical Operator2/1 -> RS FlopFlop/1(S)
  Logical Operator4/1 -> RS FlopFlop/2(R)
  EngSpd/1 -> Relational Operator7/1, Relational Operator8/1
  BatSoc/1 -> Relational Operator3/1, Relational Operator5/1
  RS FlopFlop/1(Q) -> MtrAstReq/1  "MtrAstReq"
  AstEnblSocMin_H_K/1 -> Relational Operator3/2
  VehSpd/1 -> Relational Operator4/1, Relational Operator6/1
  DrvReqTrq/1 -> Relational Operator1/1
  Brake_pedal/1 -> Relational Operator2/1
  zero/1 -> Relational Operator2/2
  Relational Operator1/1 -> Logical Operator1/1
  Relational Operator2/1 -> Logical Operator1/2
  Logical Operator1/1 -> Logical Operator3/1, Logical Operator2/1
  AstEnblSocMin_L_K/1 -> Relational Operator5/2
  AstEnblVehSpdMin_L_K/1 -> Relational Operator6/2
  AstEnblVehSpdMin_H_K/1 -> Relational Operator4/2
  AstEnblEngSpdMin_H_K/1 -> Relational Operator7/2
  Relational Operator4/1 -> Logical Operator2/2
  Relational Operator7/1 -> Logical Operator2/3
  Relational Operator3/1 -> Logical Operator2/4
  AstEnblEngSpdMin_L_K/1 -> Relational Operator8/2
  Relational Operator6/1 -> Logical Operator4/2
  Relational Operator8/1 -> Logical Operator4/3
  Logical Operator3/1 -> Logical Operator4/1
  Relational Operator5/1 -> Logical Operator4/4
  AstMinTrq/1 -> Relational Operator1/2

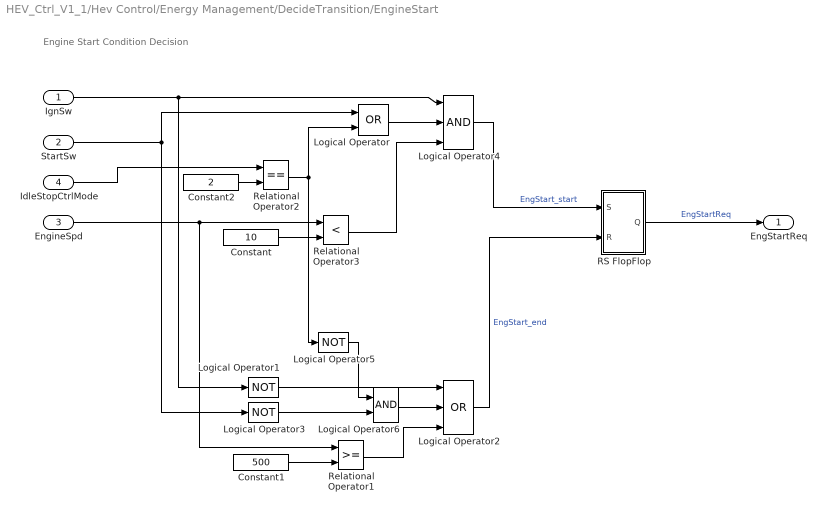
== system HEV_Ctrl_V1_1/Hev Control/Energy Management/DecideTransition/EngineStart ==
  note: Engine Start Condition Decision
  IgnSw : Inport
  StartSw : Inport  Port=2
  EngineSpd : Inport  Port=3
  IdleStopCtrlMode : Inport  Port=4
  Constant : Constant  Value=10
  Constant1 : Constant  Value=500
  Constant2 : Constant  Value=2
  Logical Operator : Logic  Operator=OR  AllPortsSameDT=off  OutDataTypeStr=boolean
  Logical Operator1 : Logic  Operator=NOT  Inputs=1  AllPortsSameDT=off  OutDataTypeStr=boolean
  Logical Operator2 : Logic  Operator=OR  Inputs=3  AllPortsSameDT=off  OutDataTypeStr=boolean
  Logical Operator3 : Logic  Operator=NOT  Inputs=1  AllPortsSameDT=off  OutDataTypeStr=boolean
  Logical Operator4 : Logic  Inputs=3  AllPortsSameDT=off  OutDataTypeStr=boolean
  Logical Operator5 : Logic  Operator=NOT  Inputs=1  AllPortsSameDT=off  OutDataTypeStr=boolean
  Logical Operator6 : Logic  AllPortsSameDT=off  OutDataTypeStr=boolean
  RS FlopFlop : Subsystem
  Relational Operator1 : RelationalOperator  OutDataTypeStr=boolean  RndMeth=Nearest
  Relational Operator2 : RelationalOperator  Operator===  OutDataTypeStr=boolean  RndMeth=Nearest
  Relational Operator3 : RelationalOperator  Operator=<  OutDataTypeStr=boolean  RndMeth=Nearest
  EngStartReq : Outport  VectorParamsAs1DForOutWhenUnconnected=off
  wires:
  IgnSw/1 -> Logical Operator1/1, Logical Operator4/1
  StartSw/1 -> Logical Operator/1, Logical Operator3/1
  EngineSpd/1 -> Relational Operator1/1, Relational Operator3/1
  Constant/1 -> Relational Operator3/2
  Relational Operator3/1 -> Logical Operator4/3
  Logical Operator3/1 -> Logical Operator6/2
  Logical Operator1/1 -> Logical Operator2/1
  Constant1/1 -> Relational Operator1/2
  Relational Operator1/1 -> Logical Operator2/3
  Logical Operator4/1 -> RS FlopFlop/1(S)  "EngStart_start"
  Logical Operator2/1 -> RS FlopFlop/2(R)  "EngStart_end"
  RS FlopFlop/1(Q) -> EngStartReq/1  "EngStartReq"
  IdleStopCtrlMode/1 -> Relational Operator2/1
  Constant2/1 -> Relational Operator2/2
  Relational Operator2/1 -> Logical Operator5/1, Logical Operator/2
  Logical Operator/1 -> Logical Operator4/2
  Logical Operator6/1 -> Logical Operator2/2
  Logical Operator5/1 -> Logical Operator6/1

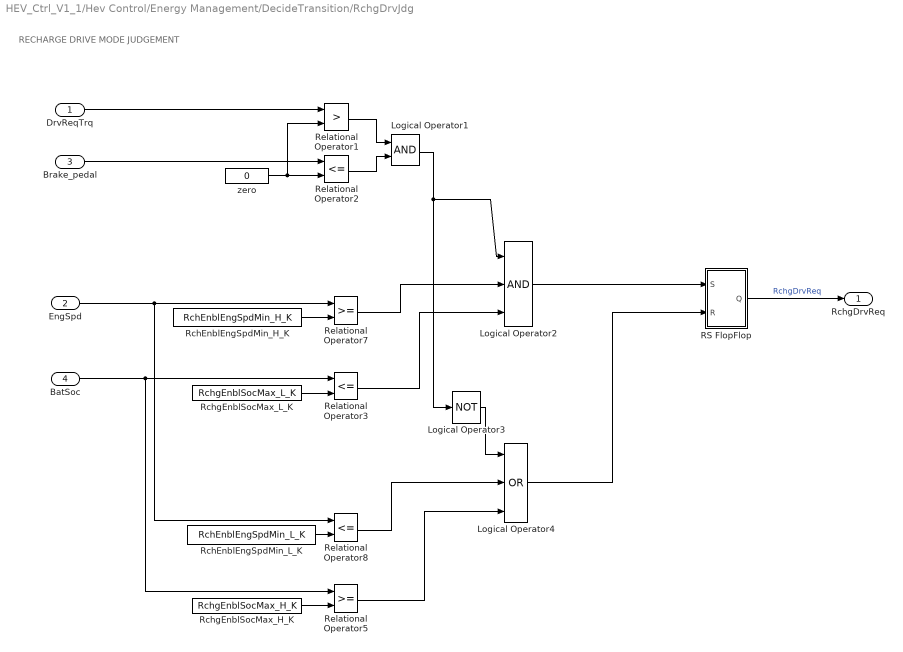
== system HEV_Ctrl_V1_1/Hev Control/Energy Management/DecideTransition/RchgDrvJdg ==
  note: RECHARGE DRIVE MODE JUDGEMENT
  DrvReqTrq : Inport
  EngSpd : Inport  Port=2
  Brake_pedal : Inport  Port=3
  BatSoc : Inport  Port=4
  Logical Operator1 : Logic  AllPortsSameDT=off  OutDataTypeStr=boolean
  Logical Operator2 : Logic  Inputs=3  AllPortsSameDT=off  OutDataTypeStr=boolean
  Logical Operator3 : Logic  Operator=NOT  AllPortsSameDT=off  OutDataTypeStr=boolean
  Logical Operator4 : Logic  Operator=OR  Inputs=3  AllPortsSameDT=off  OutDataTypeStr=boolean
  RS FlopFlop : Subsystem
  RchEnblEngSpdMin_H_K : Constant  Value=RchEnblEngSpdMin_H_K
  RchEnblEngSpdMin_L_K : Constant  Value=RchEnblEngSpdMin_L_K
  RchgEnblSocMax_H_K : Constant  Value=RchgEnblSocMax_H_K
  RchgEnblSocMax_L_K : Constant  Value=RchgEnblSocMax_L_K
  Relational Operator1 : RelationalOperator  Operator=>  OutDataTypeStr=boolean  RndMeth=Nearest
  Relational Operator2 : RelationalOperator  Operator=<=  OutDataTypeStr=boolean  RndMeth=Nearest
  Relational Operator3 : RelationalOperator  Operator=<=  OutDataTypeStr=boolean  RndMeth=Nearest
  Relational Operator5 : RelationalOperator  OutDataTypeStr=boolean  RndMeth=Nearest
  Relational Operator7 : RelationalOperator  OutDataTypeStr=boolean  RndMeth=Nearest
  Relational Operator8 : RelationalOperator  Operator=<=  OutDataTypeStr=boolean  RndMeth=Nearest
  zero : Constant  Value=0
  RchgDrvReq : Outport  VectorParamsAs1DForOutWhenUnconnected=off
  wires:
  RS FlopFlop/1(Q) -> RchgDrvReq/1  "RchgDrvReq"
  EngSpd/1 -> Relational Operator7/1, Relational Operator8/1
  BatSoc/1 -> Relational Operator3/1, Relational Operator5/1
  RchgEnblSocMax_L_K/1 -> Relational Operator3/2
  DrvReqTrq/1 -> Relational Operator1/1
  Brake_pedal/1 -> Relational Operator2/1
  zero/1 -> Relational Operator2/2, Relational Operator1/2
  Relational Operator1/1 -> Logical Operator1/1
  Relational Operator2/1 -> Logical Operator1/2
  Logical Operator1/1 -> Logical Operator3/1, Logical Operator2/1
  RchgEnblSocMax_H_K/1 -> Relational Operator5/2
  RchEnblEngSpdMin_H_K/1 -> Relational Operator7/2
  RchEnblEngSpdMin_L_K/1 -> Relational Operator8/2
  Logical Operator3/1 -> Logical Operator4/1
  Logical Operator2/1 -> RS FlopFlop/1(S)
  Relational Operator7/1 -> Logical Operator2/2
  Relational Operator3/1 -> Logical Operator2/3
  Relational Operator8/1 -> Logical Operator4/2
  Relational Operator5/1 -> Logical Operator4/3
  Logical Operator4/1 -> RS FlopFlop/2(R)

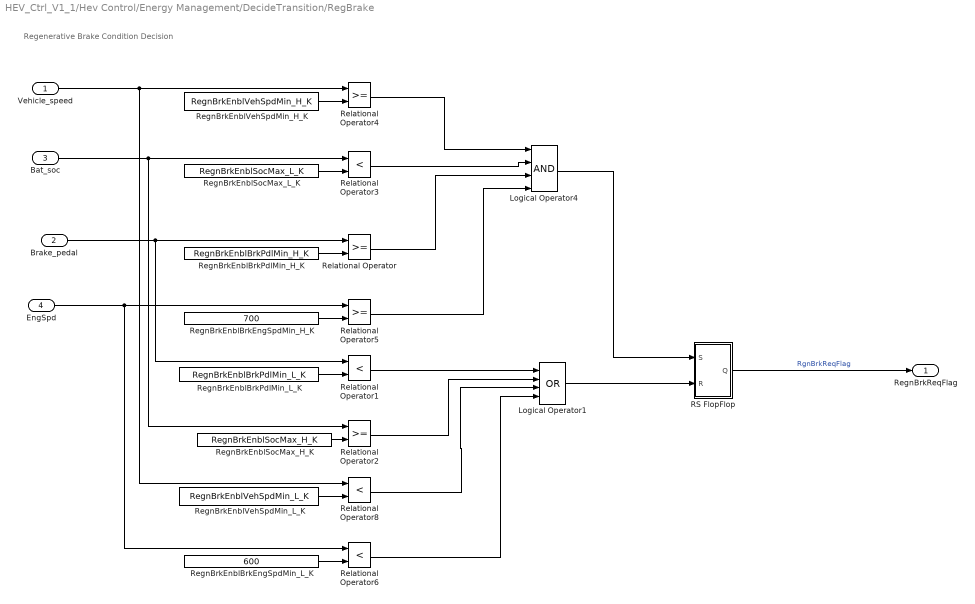
== system HEV_Ctrl_V1_1/Hev Control/Energy Management/DecideTransition/RegBrake ==
  note: Regenerative Brake Condition Decision
  Vehicle_speed : Inport
  Brake_pedal : Inport  Port=2
  Bat_soc : Inport  Port=3
  EngSpd : Inport  Port=4
  Logical Operator1 : Logic  Operator=OR  Inputs=4  AllPortsSameDT=off  OutDataTypeStr=boolean
  Logical Operator4 : Logic  Inputs=4  AllPortsSameDT=off  OutDataTypeStr=boolean
  RS FlopFlop : Subsystem
  RegnBrkEnblBrkEngSpdMin_H_K : Constant  Value=700
  RegnBrkEnblBrkEngSpdMin_L_K : Constant  Value=600
  RegnBrkEnblBrkPdlMin_H_K : Constant  Value=RegnBrkEnblBrkPdlMin_H_K
  RegnBrkEnblBrkPdlMin_L_K : Constant  Value=RegnBrkEnblBrkPdlMin_L_K
  RegnBrkEnblSocMax_H_K : Constant  Value=RegnBrkEnblSocMax_H_K
  RegnBrkEnblSocMax_L_K : Constant  Value=RegnBrkEnblSocMax_L_K
  RegnBrkEnblVehSpdMin_H_K : Constant  Value=RegnBrkEnblVehSpdMin_H_K
  RegnBrkEnblVehSpdMin_L_K : Constant  Value=RegnBrkEnblVehSpdMin_L_K
  Relational Operator{,2,4..5} (4 alike) : RelationalOperator  OutDataTypeStr=boolean  RndMeth=Nearest
  Relational Operator{1,3,6,8} (4 alike) : RelationalOperator  Operator=<  OutDataTypeStr=boolean  RndMeth=Nearest
  RegnBrkReqFlag : Outport  VectorParamsAs1DForOutWhenUnconnected=off
  wires:
  Relational Operator8/1 -> Logical Operator1/3
  Relational Operator1/1 -> Logical Operator1/1
  RegnBrkEnblVehSpdMin_L_K/1 -> Relational Operator8/2
  RegnBrkEnblBrkPdlMin_L_K/1 -> Relational Operator1/2
  Logical Operator1/1 -> RS FlopFlop/2(R)
  Relational Operator3/1 -> Logical Operator4/2
  Relational Operator4/1 -> Logical Operator4/1
  Brake_pedal/1 -> Relational Operator1/1, Relational Operator/1
  RegnBrkEnblBrkPdlMin_H_K/1 -> Relational Operator/2
  Relational Operator/1 -> Logical Operator4/3
  Bat_soc/1 -> Relational Operator3/1, Relational Operator2/1
  RegnBrkEnblSocMax_L_K/1 -> Relational Operator3/2
  RS FlopFlop/1(Q) -> RegnBrkReqFlag/1  "RgnBrkReqFlag"
  Vehicle_speed/1 -> Relational Operator8/1, Relational Operator4/1
  RegnBrkEnblVehSpdMin_H_K/1 -> Relational Operator4/2
  Logical Operator4/1 -> RS FlopFlop/1(S)
  RegnBrkEnblSocMax_H_K/1 -> Relational Operator2/2
  Relational Operator2/1 -> Logical Operator1/2
  EngSpd/1 -> Relational Operator6/1, Relational Operator5/1
  RegnBrkEnblBrkEngSpdMin_H_K/1 -> Relational Operator5/2
  Relational Operator5/1 -> Logical Operator4/4
  RegnBrkEnblBrkEngSpdMin_L_K/1 -> Relational Operator6/2
  Relational Operator6/1 -> Logical Operator1/4

== system HEV_Ctrl_V1_1/Hev Control/Energy Management/Recharge/Recharge ==
  note: Recharge
  DrvReqTrq : Inport
  EngSpd : Inport  Port=2
  MtrRgnTrqMax : Inport  Port=3
  BatSOC : Inport  Port=4
  AstTrqDstBase_K3 : Lookup2D  RowIndex=AstTrqDstBase_Y  ColumnIndex=AstTrqDstBase_X  Table=AstTrqDstBase_K3  LookUpMeth=Interpolation-Use End Values  SaturateOnIntegerOverflow=on
      settings: AttributesFormatString=<row=%<RowIndex>>\n<column=%<ColumnIndex>>
  Div : Product  Inputs=*/
  DrvReqPropTrqMax_K : Constant  Value=DrvReqPropTrqMax_K
  Gain1 : Gain  Gain=-1
  K2_EfcEngTrq : Lookup  InputValues=RchgTrqCmpSOC_X  Table=RchgTrqCmpSOC_K2  LookUpMeth=Interpolation-Use End Values  SaturateOnIntegerOverflow=on
      settings: AttributesFormatString=<input=%<InputValues>>
  MaxLimit : MinMax  Inputs=2
  Product : Product  RndMeth=Zero
  Product1 : Product  RndMeth=Zero
  Sum2 : Sum
  MtrTrqReq : Outport  VectorParamsAs1DForOutWhenUnconnected=off
  EngTrqReq : Outport  Port=2  VectorParamsAs1DForOutWhenUnconnected=off
  wires:
  DrvReqTrq/1 -> Div/1, Sum2/2, Product1/2
  K2_EfcEngTrq/1 -> Product/2
  Product/1 -> Product1/1
  BatSOC/1 -> K2_EfcEngTrq/1
  MaxLimit/1 -> Sum2/1, Gain1/1  "RchgMtrTrqReq"
  Sum2/1 -> EngTrqReq/1  "EngTrqReq"
  MtrRgnTrqMax/1 -> MaxLimit/1
  Gain1/1 -> MtrTrqReq/1  "MtrTrqReq"
  DrvReqPropTrqMax_K/1 -> Div/2
  Div/1 -> AstTrqDstBase_K3/1
  AstTrqDstBase_K3/1 -> Product/1
  EngSpd/1 -> AstTrqDstBase_K3/2
  Product1/1 -> MaxLimit/2

== system HEV_Ctrl_V1_1/Hev Control/Energy Management/RegenrativeBrake/Regenerative Brake ==
  note: MaxRegnBrkTrq = MaxRegnTrq * BRK_PROTSOC
  note: BrakeTorque @Crank Positive <--|--> Negative
  note: BrakeTorque @Crank Negaive <--|--> Positive
  note: REGENERATIVE BRAKING CO-OPERATIVE WITH FRICTION BRAKE
  MaxRegnTrq : Inport
  BattSOC : Inport  Port=2
  EbsReqMtrTrq : Inport  Port=3
  ClutchStatus : Constant
  Gain1 : Gain  Gain=-1
  Gain3 : Gain  Gain=-1
  MaxLimit : MinMax  Inputs=2
  Product2 : Product  RndMeth=Zero
  RegnBrkCmpSOC_K2 : Lookup  InputValues=RegnBrkCmpSOC_X  Table=RegnBrkCmpSOC_K2  LookUpMeth=Interpolation-Use End Values  SaturateOnIntegerOverflow=on
      settings: AttributesFormatString=<input=%<InputValues>>
  Switch1 : Switch  Criteria=u2 ~= 0  Threshold=0.5  SaturateOnIntegerOverflow=on
      settings: AttributesFormatString=<%<Criteria>>
  Switch2 : Switch  Criteria=u2 ~= 0  Threshold=0.5  SaturateOnIntegerOverflow=on
      settings: AttributesFormatString=<%<Criteria>>
  zero : Constant  Value=0
  zero1 : Constant  Value=0
  MtrTrqReq : Outport  VectorParamsAs1DForOutWhenUnconnected=off
  RegnBrkTrqMax : Outport  Port=2  VectorParamsAs1DForOutWhenUnconnected=off
  wires:
  Product2/1 -> Switch1/1  "MaxRegnBrkTrq"
  zero1/1 -> Switch1/3
  Gain3/1 -> MaxLimit/2
  EbsReqMtrTrq/1 -> Gain3/1
  Switch1/1 -> RegnBrkTrqMax/1  "RegnBrkTrqMax"
  ClutchStatus/1 -> Switch1/2, Switch2/2
  zero/1 -> Switch2/3
  MaxRegnTrq/1 -> Product2/1, MaxLimit/1
  MaxLimit/1 -> Switch2/1
  RegnBrkCmpSOC_K2/1 -> Product2/2
  BattSOC/1 -> RegnBrkCmpSOC_K2/1
  Gain1/1 -> MtrTrqReq/1  "MtrTrqReq"
  Switch2/1 -> Gain1/1

== system HEV_Ctrl_V1_1/Hev Control/Energy Management/DecideTransition/Assist/RS FlopFlop ==
  note: RS FlipFlop
  S : Inport
  R : Inport  Port=2
  false : Constant  Value=false
  if then elseif : Subsystem  mask(if then elseif){}
  true : Constant  Value=true
  Q : Outport  VectorParamsAs1DForOutWhenUnconnected=off
  wires:
  S/1 -> if then elseif/3(elseif)
  R/1 -> if then elseif/1(if)
  if then elseif/1(y) -> Q/1
  false/1 -> if then elseif/2(then1)
  true/1 -> if then elseif/4(then2)

== system HEV_Ctrl_V1_1/Hev Control/Energy Management/DecideTransition/EngineStart/RS FlopFlop ==
  note: RS FlipFlop
  S : Inport
  R : Inport  Port=2
  false : Constant  Value=false
  if then elseif : Subsystem  mask(if then elseif){}
  true : Constant  Value=true
  Q : Outport  VectorParamsAs1DForOutWhenUnconnected=off
  wires:
  true/1 -> if then elseif/4(then2)
  false/1 -> if then elseif/2(then1)
  if then elseif/1(y) -> Q/1
  R/1 -> if then elseif/1(if)
  S/1 -> if then elseif/3(elseif)

== system HEV_Ctrl_V1_1/Hev Control/Energy Management/DecideTransition/RchgDrvJdg/RS FlopFlop ==
  note: RS FlipFlop
  S : Inport
  R : Inport  Port=2
  false : Constant  Value=false
  if then elseif : Subsystem  mask(if then elseif){}
  true : Constant  Value=true
  Q : Outport  VectorParamsAs1DForOutWhenUnconnected=off
  wires:
  true/1 -> if then elseif/4(then2)
  false/1 -> if then elseif/2(then1)
  if then elseif/1(y) -> Q/1
  R/1 -> if then elseif/1(if)
  S/1 -> if then elseif/3(elseif)

== system HEV_Ctrl_V1_1/Hev Control/Energy Management/DecideTransition/RegBrake/RS FlopFlop ==
  note: RS FlipFlop
  S : Inport
  R : Inport  Port=2
  false : Constant  Value=false
  if then elseif : Subsystem  mask(if then elseif){}
  true : Constant  Value=true
  Q : Outport  VectorParamsAs1DForOutWhenUnconnected=off
  wires:
  true/1 -> if then elseif/4(then2)
  false/1 -> if then elseif/2(then1)
  if then elseif/1(y) -> Q/1
  R/1 -> if then elseif/1(if)
  S/1 -> if then elseif/3(elseif)

== system HEV_Ctrl_V1_1/Hev Control/Energy Management/DecideTransition/Assist/RS FlopFlop/if then elseif ==
  note: If then elseif
  if : Inport
  then1 : Inport  Port=2
  elseif : Inport  Port=3
  then2 : Inport  Port=4
  Data Type Conversion : DataTypeConversion  OutDataTypeStr=boolean
  Switch2 : Switch  Criteria=u2 ~= 0  Threshold=0.5  SaturateOnIntegerOverflow=on
      settings: AttributesFormatString=<%<Criteria>>
  Switch3 : Switch  Criteria=u2 ~= 0  Threshold=0.5  SaturateOnIntegerOverflow=on
      settings: AttributesFormatString=<%<Criteria>>
  Unit Delay : UnitDelay  SampleTime=-1  HasFrameUpgradeWarning=on
      settings: AttributesFormatString=<initial=%<X0>>\n<tsample=%<SampleTime>>
  y : Outport  VectorParamsAs1DForOutWhenUnconnected=off
  wires:
  Data Type Conversion/1 -> y/1
  Switch2/1 -> Switch3/3
  if/1 -> Switch3/2
  Unit Delay/1 -> Switch2/3  "y_old"
  Switch3/1 -> Data Type Conversion/1, Unit Delay/1  "y"
  then1/1 -> Switch3/1
  elseif/1 -> Switch2/2
  then2/1 -> Switch2/1

== system HEV_Ctrl_V1_1/Hev Control/Energy Management/DecideTransition/EngineStart/RS FlopFlop/if then elseif ==
  note: If then elseif
  if : Inport
  then1 : Inport  Port=2
  elseif : Inport  Port=3
  then2 : Inport  Port=4
  Data Type Conversion : DataTypeConversion  OutDataTypeStr=boolean
  Switch2 : Switch  Criteria=u2 ~= 0  Threshold=0.5  SaturateOnIntegerOverflow=on
      settings: AttributesFormatString=<%<Criteria>>
  Switch3 : Switch  Criteria=u2 ~= 0  Threshold=0.5  SaturateOnIntegerOverflow=on
      settings: AttributesFormatString=<%<Criteria>>
  Unit Delay : UnitDelay  SampleTime=-1  HasFrameUpgradeWarning=on
      settings: AttributesFormatString=<initial=%<X0>>\n<tsample=%<SampleTime>>
  y : Outport  VectorParamsAs1DForOutWhenUnconnected=off
  wires:
  then2/1 -> Switch2/1
  elseif/1 -> Switch2/2
  then1/1 -> Switch3/1
  Switch3/1 -> Unit Delay/1, Data Type Conversion/1  "y"
  Unit Delay/1 -> Switch2/3  "y_old"
  if/1 -> Switch3/2
  Switch2/1 -> Switch3/3
  Data Type Conversion/1 -> y/1

== system HEV_Ctrl_V1_1/Hev Control/Energy Management/DecideTransition/RchgDrvJdg/RS FlopFlop/if then elseif ==
  note: If then elseif
  if : Inport
  then1 : Inport  Port=2
  elseif : Inport  Port=3
  then2 : Inport  Port=4
  Data Type Conversion : DataTypeConversion  OutDataTypeStr=boolean
  Switch2 : Switch  Criteria=u2 ~= 0  Threshold=0.5  SaturateOnIntegerOverflow=on
      settings: AttributesFormatString=<%<Criteria>>
  Switch3 : Switch  Criteria=u2 ~= 0  Threshold=0.5  SaturateOnIntegerOverflow=on
      settings: AttributesFormatString=<%<Criteria>>
  Unit Delay : UnitDelay  SampleTime=-1  HasFrameUpgradeWarning=on
      settings: AttributesFormatString=<initial=%<X0>>\n<tsample=%<SampleTime>>
  y : Outport  VectorParamsAs1DForOutWhenUnconnected=off
  wires:
  then2/1 -> Switch2/1
  elseif/1 -> Switch2/2
  then1/1 -> Switch3/1
  Switch3/1 -> Unit Delay/1, Data Type Conversion/1  "y"
  Unit Delay/1 -> Switch2/3  "y_old"
  if/1 -> Switch3/2
  Switch2/1 -> Switch3/3
  Data Type Conversion/1 -> y/1

== system HEV_Ctrl_V1_1/Hev Control/Energy Management/DecideTransition/RegBrake/RS FlopFlop/if then elseif ==
  note: If then elseif
  if : Inport
  then1 : Inport  Port=2
  elseif : Inport  Port=3
  then2 : Inport  Port=4
  Data Type Conversion : DataTypeConversion  OutDataTypeStr=boolean
  Switch2 : Switch  Criteria=u2 ~= 0  Threshold=0.5  SaturateOnIntegerOverflow=on
      settings: AttributesFormatString=<%<Criteria>>
  Switch3 : Switch  Criteria=u2 ~= 0  Threshold=0.5  SaturateOnIntegerOverflow=on
      settings: AttributesFormatString=<%<Criteria>>
  Unit Delay : UnitDelay  SampleTime=-1  HasFrameUpgradeWarning=on
      settings: AttributesFormatString=<initial=%<X0>>\n<tsample=%<SampleTime>>
  y : Outport  VectorParamsAs1DForOutWhenUnconnected=off
  wires:
  then2/1 -> Switch2/1
  elseif/1 -> Switch2/2
  then1/1 -> Switch3/1
  Switch3/1 -> Unit Delay/1, Data Type Conversion/1  "y"
  Unit Delay/1 -> Switch2/3  "y_old"
  if/1 -> Switch3/2
  Switch2/1 -> Switch3/3
  Data Type Conversion/1 -> y/1
